simulink model "moyenneur"  (R2019a)
settings: Solver=VariableStepAuto  StartTime=0.0  StopTime=30  RelTol=1e-3
libraries: Librairie x2
settings Model: Creator=shse  LastModifiedBy=shse

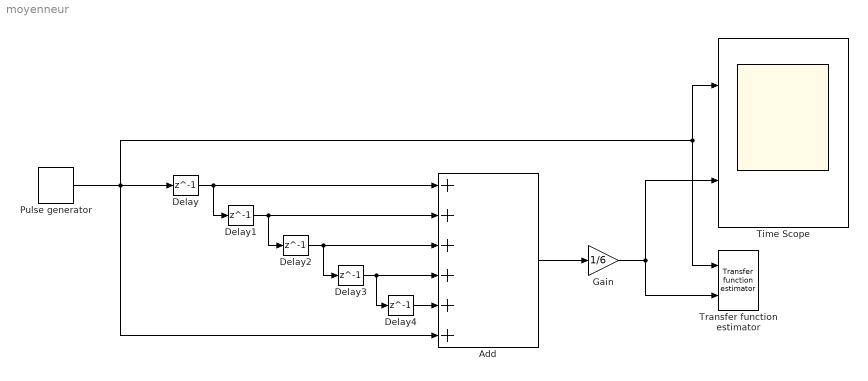
== system moyenneur ==
  Add : Sum  Inputs=++++++
  Delay{,1..4} (5 alike) : Delay  DelayLength=1  InitialCondition=0  InputProcessing=Columns as channels (frame based)
  Gain : Gain  Gain=1/6
  Pulse generator : Librairie/Pulse generator  fee=11025  NN=1024
  Time Scope : Scope  NumInputPorts=2
  Transfer function estimator : Librairie/Transfer function estimator  fee=11025  NN=1024
  wires:
  Delay/1 -> Delay1/1, Add/1
  Add/1 -> Gain/1
  Pulse generator/1 -> Delay/1, Add/6, Transfer function estimator/1, Time Scope/1
  Gain/1 -> Time Scope/2, Transfer function estimator/2
  Delay1/1 -> Delay2/1, Add/2
  Delay2/1 -> Add/3, Delay3/1
  Delay3/1 -> Add/4, Delay4/1
  Delay4/1 -> Add/5
